simulink model "Sistema"  (R2023a)
settings: Solver=ode15s  StartTime=0.0  StopTime=10.0  MaxStep=1E-3  RelTol=1e-3
libraries: fl_lib x21, nesl_utility x9, slpidlib x2
settings Model: Creator=lunit  LastModifiedBy=Dino
settings DataIOCC: SaveFormat=Array  ReturnWorkspaceOutputs=off  TimeSaveName=t
settings DebuggingCC: AlgebraicLoopMsg=none  ArtificialAlgebraicLoopMsg=none  MaxConsecutiveZCsMsg=none  UnconnectedInputMsg=warning  UnconnectedOutputMsg=warning  UnconnectedLineMsg=warning  ModelReferenceExtraNoncontSigs=none  OperatingPointInterfaceChecksumMismatchMsg=none
settings ModelReferenceCC: EnableRefExpFcnMdlSchedulingChecks=on
settings RTWCC: DLArmComputeVersion=19.05

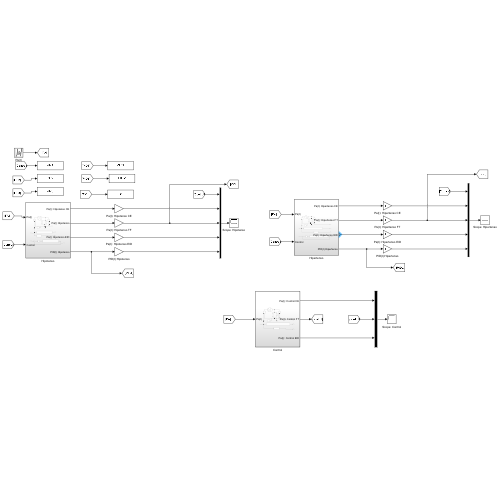
[thumbnail: Simulink's stored preview of the top-level diagram]
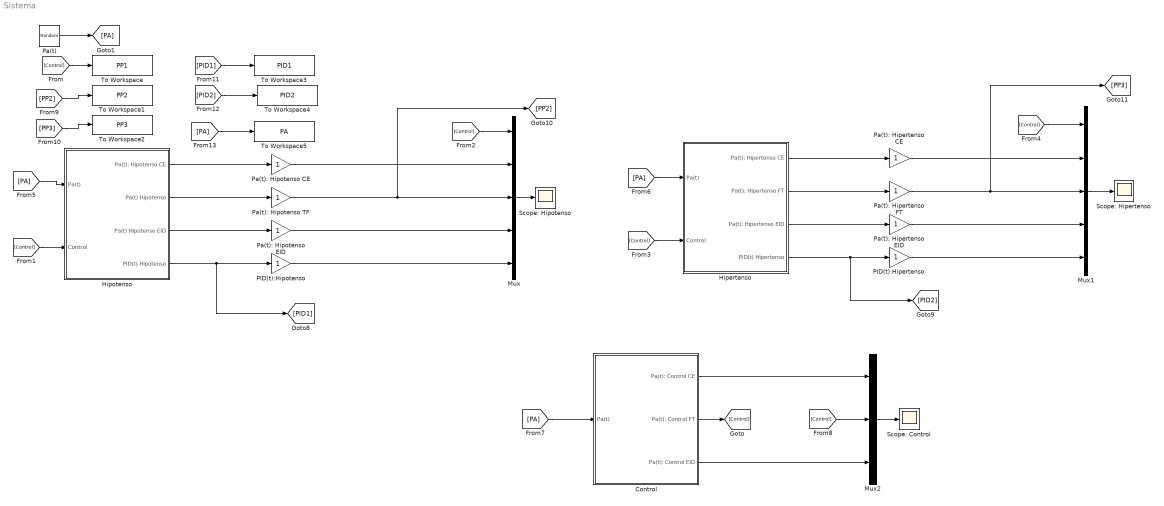
== system Sistema ==
  Control : Subsystem
  Hipertenso : Subsystem
  Hipotenso : Subsystem
  Mux : Mux  Inputs=5
  Mux1 : Mux  Inputs=5
  Mux2 : Mux  Inputs=3
  PID(t):Hipertenso : Gain
  PID(t):Hipotenso : Gain
  Pa(t) : UniformRandomNumber  Minimum=-0.2  Seed=106  SampleTime=0.5
  Pa(t): Hipertenso CE : Gain
  Pa(t): Hipertenso EID : Gain
  Pa(t): Hipertenso FT : Gain
  Pa(t): Hipotenso CE : Gain
  Pa(t): Hipotenso EID : Gain
  Pa(t): Hipotenso TF : Gain
  Scope: Control : Scope
  Scope: Hipertenso : Scope
  Scope: Hipotenso : Scope
  To Workspace : ToWorkspace  VariableName=PP1  SampleTime=-1
  To Workspace1 : ToWorkspace  VariableName=PP2  SampleTime=-1
  To Workspace2 : ToWorkspace  VariableName=PP3  SampleTime=-1
  To Workspace3 : ToWorkspace  VariableName=PID1  SampleTime=-1
  To Workspace4 : ToWorkspace  VariableName=PID2  SampleTime=-1
  To Workspace5 : ToWorkspace  VariableName=PA  SampleTime=-1
  wires:
  Mux/1 -> Scope: Hipotenso/1
  Hipotenso/1(Pa(t): Hipotenso CE) -> Pa(t): Hipotenso CE/1
  Hipotenso/2(Pa(t) Hipotenso) -> Pa(t): Hipotenso TF/1
  Hipotenso/3(Pa(t) Hipotenso EID) -> Pa(t): Hipotenso EID/1
  Hipotenso/4(PID(t) Hipotenso) -> [PID1], PID(t):Hipotenso/1
  [Control] -> Mux/1
  Pa(t): Hipotenso CE/1 -> Mux/2
  PID(t):Hipotenso/1 -> Mux/5
  Pa(t): Hipotenso EID/1 -> Mux/4
  Pa(t): Hipotenso TF/1 -> [PP2], Mux/3
  [Control] -> Hipotenso/2(Control)
  Pa(t): Hipertenso FT/1 -> [PP3], Mux1/3
  PID(t):Hipertenso/1 -> Mux1/5
  Mux1/1 -> Scope: Hipertenso/1
  Hipertenso/3(Pa(t): Hipertenso EID) -> Pa(t): Hipertenso EID/1
  Hipertenso/1(Pa(t): Hipertenso CE) -> Pa(t): Hipertenso CE/1
  Hipertenso/4(PID(t) Hipertenso) -> [PID2], PID(t):Hipertenso/1
  Pa(t): Hipertenso CE/1 -> Mux1/2
  Pa(t): Hipertenso EID/1 -> Mux1/4
  [Control] -> Mux1/1
  Hipertenso/2(Pa(t): Hipertenso FT) -> Pa(t): Hipertenso FT/1
  [Control] -> Hipertenso/2(Control)
  Pa(t)/1 -> [PA]
  [PA] -> Hipotenso/1(Pa(t))
  [PA] -> Hipertenso/1(Pa(t))
  Control/2(Pa(t): Control FT) -> [Control]
  [PA] -> Control/1(Pa(t))
  Mux2/1 -> Scope: Control/1
  Control/3(Pa(t): Control EID) -> Mux2/3
  Control/1(Pa(t): Control CE) -> Mux2/1
  [Control] -> Mux2/2
  [Control] -> To Workspace/1
  [PP2] -> To Workspace1/1
  [PP3] -> To Workspace2/1
  [PID1] -> To Workspace3/1
  [PID2] -> To Workspace4/1
  [PA] -> To Workspace5/1

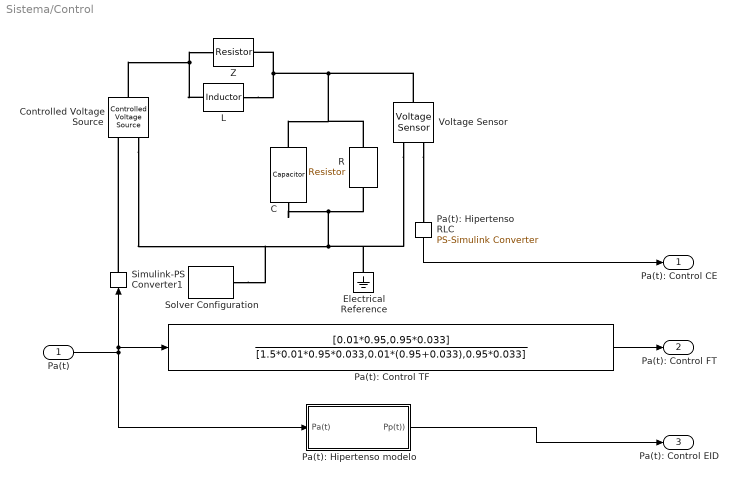
== system Sistema/Control ==
  Pa(t) : Inport
  C : fl_lib/Electrical/Electrical Elements/Capacitor  c=1.5 F  r=1e-6 Ohm  g=0 1/Ohm  i_specify=off  i_priority=None  i=0 A  i_nominal_specify=off  i_nominal_unit=A  i_nominal_value=1  v_specify=off  v_priority=None  v=0 V  v_nominal_specify=off  v_nominal_unit=V  v_nominal_value=1  vc_specify=off  vc_priority=High  vc=0 V  vc_nominal_specify=off  vc_nominal_unit=V  vc_nominal_value=1
  Controlled Voltage Source : fl_lib/Electrical/Electrical Sources/Controlled Voltage Source
  Electrical Reference : fl_lib/Electrical/Electrical Elements/Electrical Reference
  L : fl_lib/Electrical/Electrical Elements/Inductor  l=0.01 H  r=0 Ohm  g=1e-9 1/Ohm  i_specify=off  i_priority=None  i=0 A  i_nominal_specify=off  i_nominal_unit=A  i_nominal_value=1  v_specify=off  v_priority=None  v=0 V  v_nominal_specify=off  v_nominal_unit=V  v_nominal_value=1  i_L_specify=off  i_L_priority=High  i_L=0 A  i_L_nominal_specify=off  i_L_nominal_unit=A  i_L_nominal_value=1
  Pa(t): Control TF : TransferFcn  Numerator=[0.01*0.95,0.95*0.033]  Denominator=[1.5*0.01*0.95*0.033,0.01*(0.95+0.033),0.95*0.033]
  Pa(t): Hipertenso RLC : nesl_utility/PS-Simulink Converter  PhysicalDomain=network_engine_domain  SubClassName=ps_output  LeftPortType=input  RightPortType=output  PseudoPeriodic=off  Frequencies=[]  VectorFormat=1-D array  Unit=inherit  AffineConversion=off
  Pa(t): Hipertenso modelo : Subsystem
  R : fl_lib/Electrical/Electrical Elements/Resistor  R=0.95 Ohm  i_specify=off  i_priority=None  i=0 A  i_nominal_specify=off  i_nominal_unit=A  i_nominal_value=1  v_specify=off  v_priority=None  v=0 V  v_nominal_specify=off  v_nominal_unit=V  v_nominal_value=1
  Simulink-PS Converter1 : nesl_utility/Simulink-PS Converter  PhysicalDomain=network_engine_domain  SubClassName=ps_input  LeftPortType=input  RightPortType=output  PseudoPeriodic=off  Frequencies=[]  NoiseDistribution=none  NoiseParameters=[]  Unit=1  AffineConversion=off  FilteringAndDerivatives=provide  SimscapeFilterOrder=1  InputFilterTimeConstant=0.001  UdotUserProvided=0
  Solver Configuration : nesl_utility/Solver Configuration  PhysicalDomain=network_engine_domain  SubClassName=solver  LeftPortType=input  RightPortType=generic  Tones=[]  Harmonics=[]  SimulateNoise=off  Profile=off  UseLocalSampling=off  EnableSwitchedLinearOptims=on  FrequencyDomain=off  UseCCode=off  RelTol=0.001  AbsTol=1e-06  MinStep=1e-09  ToWorkspace=off  RevertToSquareIcSolve=off  NumHomotopyIterations=100  PhasorMode=off  PhasorModeNumHarmonics=1  ConsistencySolver=NEWTON_FTOL  IndexReductionMethod=DerivativeReplacement  DoDC=off  ResidualTolerance=1e-09  ConsistencyTolSource=GLOBAL  ConsistencyAbsTol=0.001  ConsistencyRelTol=0.001  ConsistencyTolFactor=0.001  UseLocalSolver=off  LocalSolverChoice=NE_BACKWARD_EULER_ADVANCER  ResolveIndetEquations=on  FunctionEvalNumThread=1  LocalSolverSampleTime=0.001  DoFixedCost=off  MaxNonlinIter=3  MaxModeIter=2  ComputeImpulses=off  ImpulseIterations=2  LinearAlgebra=auto  LinearAlgebraNumThread=0  EquationFormulation=NE_TIME_EF  DelaysMemoryBudget=1024  AutomaticFiltering=on  FilteringTimeConstant=0.001  PartitionStorageMethod=AS_NEEDED  PartitionMemoryBudget=1024  PartitionMethod=ROBUST
  Voltage Sensor : fl_lib/Electrical/Electrical Sensors/Voltage Sensor
  Z : fl_lib/Electrical/Electrical Elements/Resistor  R=0.033 Ohm  i_specify=off  i_priority=None  i=0 A  i_nominal_specify=off  i_nominal_unit=A  i_nominal_value=1  v_specify=off  v_priority=None  v=0 V  v_nominal_specify=off  v_nominal_unit=V  v_nominal_value=1
  Pa(t): Control CE : Outport
  Pa(t): Control FT : Outport  Port=2
  Pa(t): Control EID : Outport  Port=3
  wires:
  Pa(t)/1 -> Pa(t): Hipertenso modelo/1(Pa(t)), Pa(t): Control TF/1, Simulink-PS Converter1/1
  Pa(t): Hipertenso RLC/1 -> Pa(t): Control CE/1
  Pa(t): Hipertenso modelo/1(Pp(t))) -> Pa(t): Control EID/1
  Pa(t): Control TF/1 -> Pa(t): Control FT/1
  connections:
  Voltage Sensor/RConn1 -- Pa(t): Hipertenso RLC/LConn1
  Simulink-PS Converter1/RConn1 -- Controlled Voltage Source/RConn1
  Controlled Voltage Source/LConn1 -- L/LConn1 -- Z/LConn1
  L/RConn1 -- Z/RConn1 -- Voltage Sensor/LConn1 -- R/LConn1 -- C/LConn1
  C/RConn1 -- Electrical Reference/LConn1 -- Voltage Sensor/RConn2 -- Controlled Voltage Source/RConn2 -- Solver Configuration/RConn1 -- R/RConn1

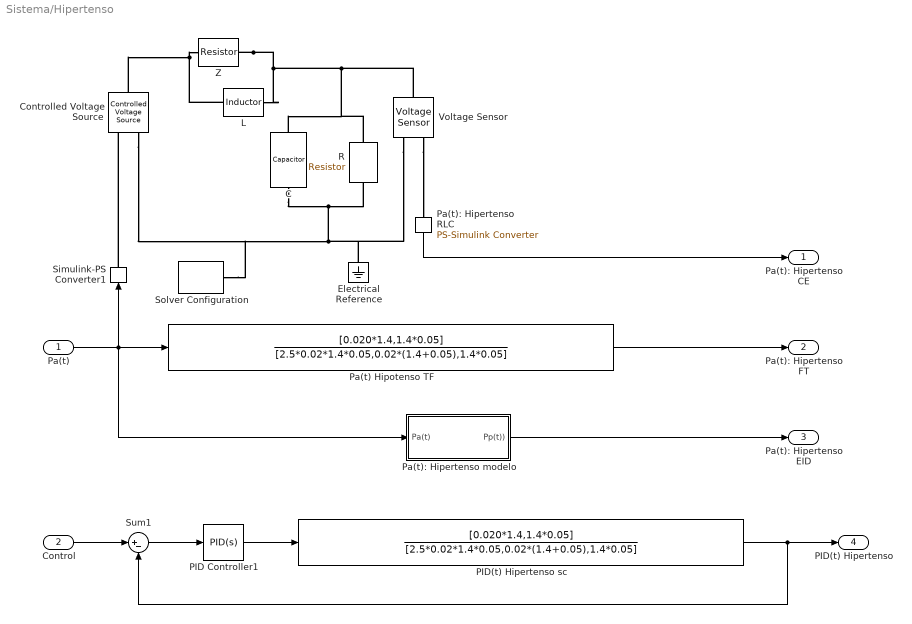
== system Sistema/Hipertenso ==
  Pa(t) : Inport
  Control : Inport  Port=2
  C : fl_lib/Electrical/Electrical Elements/Capacitor  c=2.5 F  r=1e-6 Ohm  g=0 1/Ohm  i_specify=off  i_priority=None  i=0 A  i_nominal_specify=off  i_nominal_unit=A  i_nominal_value=1  v_specify=off  v_priority=None  v=0 V  v_nominal_specify=off  v_nominal_unit=V  v_nominal_value=1  vc_specify=off  vc_priority=High  vc=0 V  vc_nominal_specify=off  vc_nominal_unit=V  vc_nominal_value=1
  Controlled Voltage Source : fl_lib/Electrical/Electrical Sources/Controlled Voltage Source
  Electrical Reference : fl_lib/Electrical/Electrical Elements/Electrical Reference
  L : fl_lib/Electrical/Electrical Elements/Inductor  l=0.02 H  r=0 Ohm  g=1e-9 1/Ohm  i_specify=off  i_priority=None  i=0 A  i_nominal_specify=off  i_nominal_unit=A  i_nominal_value=1  v_specify=off  v_priority=None  v=0 V  v_nominal_specify=off  v_nominal_unit=V  v_nominal_value=1  i_L_specify=off  i_L_priority=High  i_L=0 A  i_L_nominal_specify=off  i_L_nominal_unit=A  i_L_nominal_value=1
  PID Controller1 : slpidlib/PID Controller  Controller=PID  Form=Parallel  TimeDomain=Continuous-time  UseExternalTs=off  SampleTime=-1  IntegratorMethod=Forward Euler  FilterMethod=Forward Euler  ControllerParametersSource=internal  P=5.71697910151292  I=98.3466226969931  UseKiTs=off  D=0.0309945192714663  N=88.3932329939867  UseFilter=on  TunerSelectOption=Transfer Function Based (PID Tuner App)  InitialConditionSource=internal  InitialConditionForIntegrator=0  InitialConditionForFilter=0  DifferentiatorICPrevScaledInput=0  ExternalReset=none  TrackingMode=off  Kt=1  LimitOutput=off  SatLimitsSource=internal  UpperSaturationLimit=inf  LowerSaturationLimit=-inf  LinearizeAsGain=on  AntiWindupMode=none  Kb=1  LimitIntegrator=off  UpperIntegratorSaturationLimit=inf  LowerIntegratorSaturationLimit=-inf  POutMin=[]  POutMax=[]  IOutMin=[]  IOutMax=[]  DOutMin=[]  DOutMax=[]  NOutMin=[]  NOutMax=[]  SumOutMin=[]  SumOutMax=[]  SaturationOutMin=[]  SaturationOutMax=[]  PParamMin=[]  PParamMax=[]  IParamMin=[]  IParamMax=[]  DParamMin=[]  DParamMax=[]  NParamMin=[]  NParamMax=[]  KbParamMin=[]  KbParamMax=[]  KtParamMin=[]  KtParamMax=[]  KbOutMin=[]  KbOutMax=[]  KtOutMin=[]  KtOutMax=[]  IntegratorOutMin=[]  IntegratorOutMax=[]  FilterOutMin=[]  FilterOutMax=[]  SumI1OutMin=[]  SumI1OutMax=[]  SumI2OutMin=[]  SumI2OutMax=[]  SumI3OutMin=[]  SumI3OutMax=[]  SumI4OutMin=[]  SumI4OutMax=[]  SumDOutMin=[]  SumDOutMax=[]  DifferentiatorOutMin=[]  DifferentiatorOutMax=[]  FilterDiffOutCoefMin=[]  FilterDiffOutCoefMax=[]  ReciprocalOutMin=[]  ReciprocalOutMax=[]  SumDenOutMin=[]  SumDenOutMax=[]  SumNumOutMin=[]  SumNumOutMax=[]  DivideOutMin=[]  DivideOutMax=[]  UdiffTsProdOutMin=[]  UdiffTsProdOutMax=[]  NTsProdOutMin=[]  NTsProdOutMax=[]  UintegralTsProdOutMin=[]  UintegralTsProdOutMax=[]  UngainTsProdOutMin=[]  UngainTsProdOutMax=[]  ClampingZeroOutDataTypeStr=Inherit: Inherit via back propagation  ClampingZeroOutMin=[]  ClampingZeroOutMax=[]  FilterDenConstantOutDataTypeStr=Inherit: Inherit via back propagation  FilterDenConstantOutMin=[]  FilterDenConstantOutMax=[]  PCopyOutDataTypeStr=Inherit: Inherit via back propagation  PCopyOutMin=[]  PCopyOutMax=[]  NCopyOutDataTypeStr=Inherit: Inherit via back propagation  NCopyOutMin=[]  NCopyOutMax=[]  IntegratorContinuousStateAttributes=''  IntegratorStateMustResolveToSignalObject=off  IntegratorRTWStateStorageClass=Auto  FilterContinuousStateAttributes=''  FilterStateMustResolveToSignalObject=off  FilterRTWStateStorageClass=Auto  ParallelPVariant=InternalParameters  IdealPVariant=Disabled  IVariant=InternalParameters  DVariant=InternalParameters  IntegratorVariant=Continuous  SatVariant=Disabled  AWVariant=Passthrough  PCopyVariant=Disabled  TRVariant=Disabled  FdbkBlocksVariant=Forward  IdealPFdbkVariant=Disabled  SatFdbkVariant=Disabled  DerivativeFilterVariant=ContFilter  NVariant=InternalParameters  NCopyVariant=Disabled  FilterICVariant=InternalICsFilter  IntegratorICVariant=InternalICs  ExternalResetVariant=Disabled  TRSumVariant=Passthrough  SumFdbkVariant=Disabled  SumVariant=Sum_PID  TsampFilterVariant=InternalTs  TsampNgainVariant=Passthrough  TsampIntegralVariant=Disabled_SignalSpec  ExternalSaturationOutDataTypeStr=Inherit: Same as second input
  PID(t) Hipertenso sc : TransferFcn  Numerator=[0.020*1.4,1.4*0.05]  Denominator=[2.5*0.02*1.4*0.05,0.02*(1.4+0.05),1.4*0.05]
  Pa(t) Hipotenso TF : TransferFcn  Numerator=[0.020*1.4,1.4*0.05]  Denominator=[2.5*0.02*1.4*0.05,0.02*(1.4+0.05),1.4*0.05]
  Pa(t): Hipertenso RLC : nesl_utility/PS-Simulink Converter  PhysicalDomain=network_engine_domain  SubClassName=ps_output  LeftPortType=input  RightPortType=output  PseudoPeriodic=off  Frequencies=[]  VectorFormat=1-D array  Unit=inherit  AffineConversion=off
  Pa(t): Hipertenso modelo : Subsystem
  R : fl_lib/Electrical/Electrical Elements/Resistor  R=1.4 Ohm  i_specify=off  i_priority=None  i=0 A  i_nominal_specify=off  i_nominal_unit=A  i_nominal_value=1  v_specify=off  v_priority=None  v=0 V  v_nominal_specify=off  v_nominal_unit=V  v_nominal_value=1
  Simulink-PS Converter1 : nesl_utility/Simulink-PS Converter  PhysicalDomain=network_engine_domain  SubClassName=ps_input  LeftPortType=input  RightPortType=output  PseudoPeriodic=off  Frequencies=[]  NoiseDistribution=none  NoiseParameters=[]  Unit=1  AffineConversion=off  FilteringAndDerivatives=provide  SimscapeFilterOrder=1  InputFilterTimeConstant=0.001  UdotUserProvided=0
  Solver Configuration : nesl_utility/Solver Configuration  PhysicalDomain=network_engine_domain  SubClassName=solver  LeftPortType=input  RightPortType=generic  Tones=[]  Harmonics=[]  SimulateNoise=off  Profile=off  UseLocalSampling=off  EnableSwitchedLinearOptims=on  FrequencyDomain=off  UseCCode=off  RelTol=0.001  AbsTol=1e-06  MinStep=1e-09  ToWorkspace=off  RevertToSquareIcSolve=off  NumHomotopyIterations=100  PhasorMode=off  PhasorModeNumHarmonics=1  ConsistencySolver=NEWTON_FTOL  IndexReductionMethod=DerivativeReplacement  DoDC=off  ResidualTolerance=1e-09  ConsistencyTolSource=GLOBAL  ConsistencyAbsTol=0.001  ConsistencyRelTol=0.001  ConsistencyTolFactor=0.001  UseLocalSolver=off  LocalSolverChoice=NE_BACKWARD_EULER_ADVANCER  ResolveIndetEquations=on  FunctionEvalNumThread=1  LocalSolverSampleTime=0.001  DoFixedCost=off  MaxNonlinIter=3  MaxModeIter=2  ComputeImpulses=off  ImpulseIterations=2  LinearAlgebra=auto  LinearAlgebraNumThread=0  EquationFormulation=NE_TIME_EF  DelaysMemoryBudget=1024  AutomaticFiltering=on  FilteringTimeConstant=0.001  PartitionStorageMethod=AS_NEEDED  PartitionMemoryBudget=1024  PartitionMethod=ROBUST
  Sum1 : Sum  Inputs=|+-
  Voltage Sensor : fl_lib/Electrical/Electrical Sensors/Voltage Sensor
  Z : fl_lib/Electrical/Electrical Elements/Resistor  R=0.05 Ohm  i_specify=off  i_priority=None  i=0 A  i_nominal_specify=off  i_nominal_unit=A  i_nominal_value=1  v_specify=off  v_priority=None  v=0 V  v_nominal_specify=off  v_nominal_unit=V  v_nominal_value=1
  Pa(t): Hipertenso CE : Outport
  Pa(t): Hipertenso FT : Outport  Port=2
  Pa(t): Hipertenso EID : Outport  Port=3
  PID(t) Hipertenso : Outport  Port=4
  wires:
  PID Controller1/1 -> PID(t) Hipertenso sc/1
  Sum1/1 -> PID Controller1/1
  PID(t) Hipertenso sc/1 -> Sum1/2, PID(t) Hipertenso/1
  Pa(t)/1 -> Pa(t) Hipotenso TF/1, Pa(t): Hipertenso modelo/1(Pa(t)), Simulink-PS Converter1/1
  Pa(t) Hipotenso TF/1 -> Pa(t): Hipertenso FT/1
  Pa(t): Hipertenso RLC/1 -> Pa(t): Hipertenso CE/1
  Control/1 -> Sum1/1
  Pa(t): Hipertenso modelo/1(Pp(t))) -> Pa(t): Hipertenso EID/1
  connections:
  Voltage Sensor/RConn1 -- Pa(t): Hipertenso RLC/LConn1
  Simulink-PS Converter1/RConn1 -- Controlled Voltage Source/RConn1
  Controlled Voltage Source/LConn1 -- L/LConn1 -- Z/LConn1
  Z/RConn1 -- L/RConn1 -- Voltage Sensor/LConn1 -- C/LConn1 -- R/LConn1
  C/RConn1 -- Electrical Reference/LConn1 -- Voltage Sensor/RConn2 -- Controlled Voltage Source/RConn2 -- Solver Configuration/RConn1 -- R/RConn1

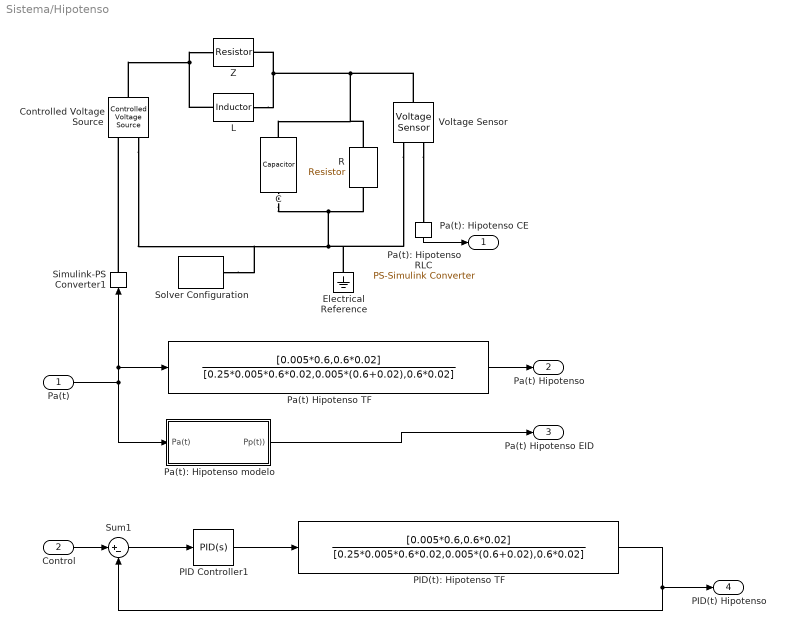
== system Sistema/Hipotenso ==
  Pa(t) : Inport
  Control : Inport  Port=2
  C : fl_lib/Electrical/Electrical Elements/Capacitor  c=0.25 F  r=1e-6 Ohm  g=0 1/Ohm  i_specify=off  i_priority=None  i=0 A  i_nominal_specify=off  i_nominal_unit=A  i_nominal_value=1  v_specify=off  v_priority=None  v=0 V  v_nominal_specify=off  v_nominal_unit=V  v_nominal_value=1  vc_specify=off  vc_priority=High  vc=0 V  vc_nominal_specify=off  vc_nominal_unit=V  vc_nominal_value=1
  Controlled Voltage Source : fl_lib/Electrical/Electrical Sources/Controlled Voltage Source
  Electrical Reference : fl_lib/Electrical/Electrical Elements/Electrical Reference
  L : fl_lib/Electrical/Electrical Elements/Inductor  l=0.005 H  r=0 Ohm  g=1e-9 1/Ohm  i_specify=off  i_priority=None  i=0 A  i_nominal_specify=off  i_nominal_unit=A  i_nominal_value=1  v_specify=off  v_priority=None  v=0 V  v_nominal_specify=off  v_nominal_unit=V  v_nominal_value=1  i_L_specify=off  i_L_priority=High  i_L=0 A  i_L_nominal_specify=off  i_L_nominal_unit=A  i_L_nominal_value=1
  PID Controller1 : slpidlib/PID Controller  Controller=PID  Form=Parallel  TimeDomain=Continuous-time  UseExternalTs=off  SampleTime=-1  IntegratorMethod=Forward Euler  FilterMethod=Forward Euler  ControllerParametersSource=internal  P=1.31715584559549  I=295.122019144814  UseKiTs=off  D=0.000356490864198976  N=467.636469275933  UseFilter=on  TunerSelectOption=Transfer Function Based (PID Tuner App)  InitialConditionSource=internal  InitialConditionForIntegrator=0  InitialConditionForFilter=0  DifferentiatorICPrevScaledInput=0  ExternalReset=none  TrackingMode=off  Kt=1  LimitOutput=off  SatLimitsSource=internal  UpperSaturationLimit=inf  LowerSaturationLimit=-inf  LinearizeAsGain=on  AntiWindupMode=none  Kb=1  LimitIntegrator=off  UpperIntegratorSaturationLimit=inf  LowerIntegratorSaturationLimit=-inf  POutMin=[]  POutMax=[]  IOutMin=[]  IOutMax=[]  DOutMin=[]  DOutMax=[]  NOutMin=[]  NOutMax=[]  SumOutMin=[]  SumOutMax=[]  SaturationOutMin=[]  SaturationOutMax=[]  PParamMin=[]  PParamMax=[]  IParamMin=[]  IParamMax=[]  DParamMin=[]  DParamMax=[]  NParamMin=[]  NParamMax=[]  KbParamMin=[]  KbParamMax=[]  KtParamMin=[]  KtParamMax=[]  KbOutMin=[]  KbOutMax=[]  KtOutMin=[]  KtOutMax=[]  IntegratorOutMin=[]  IntegratorOutMax=[]  FilterOutMin=[]  FilterOutMax=[]  SumI1OutMin=[]  SumI1OutMax=[]  SumI2OutMin=[]  SumI2OutMax=[]  SumI3OutMin=[]  SumI3OutMax=[]  SumI4OutMin=[]  SumI4OutMax=[]  SumDOutMin=[]  SumDOutMax=[]  DifferentiatorOutMin=[]  DifferentiatorOutMax=[]  FilterDiffOutCoefMin=[]  FilterDiffOutCoefMax=[]  ReciprocalOutMin=[]  ReciprocalOutMax=[]  SumDenOutMin=[]  SumDenOutMax=[]  SumNumOutMin=[]  SumNumOutMax=[]  DivideOutMin=[]  DivideOutMax=[]  UdiffTsProdOutMin=[]  UdiffTsProdOutMax=[]  NTsProdOutMin=[]  NTsProdOutMax=[]  UintegralTsProdOutMin=[]  UintegralTsProdOutMax=[]  UngainTsProdOutMin=[]  UngainTsProdOutMax=[]  ClampingZeroOutDataTypeStr=Inherit: Inherit via back propagation  ClampingZeroOutMin=[]  ClampingZeroOutMax=[]  FilterDenConstantOutDataTypeStr=Inherit: Inherit via back propagation  FilterDenConstantOutMin=[]  FilterDenConstantOutMax=[]  PCopyOutDataTypeStr=Inherit: Inherit via back propagation  PCopyOutMin=[]  PCopyOutMax=[]  NCopyOutDataTypeStr=Inherit: Inherit via back propagation  NCopyOutMin=[]  NCopyOutMax=[]  IntegratorContinuousStateAttributes=''  IntegratorStateMustResolveToSignalObject=off  IntegratorRTWStateStorageClass=Auto  FilterContinuousStateAttributes=''  FilterStateMustResolveToSignalObject=off  FilterRTWStateStorageClass=Auto  ParallelPVariant=InternalParameters  IdealPVariant=Disabled  IVariant=InternalParameters  DVariant=InternalParameters  IntegratorVariant=Continuous  SatVariant=Disabled  AWVariant=Passthrough  PCopyVariant=Disabled  TRVariant=Disabled  FdbkBlocksVariant=Forward  IdealPFdbkVariant=Disabled  SatFdbkVariant=Disabled  DerivativeFilterVariant=ContFilter  NVariant=InternalParameters  NCopyVariant=Disabled  FilterICVariant=InternalICsFilter  IntegratorICVariant=InternalICs  ExternalResetVariant=Disabled  TRSumVariant=Passthrough  SumFdbkVariant=Disabled  SumVariant=Sum_PID  TsampFilterVariant=InternalTs  TsampNgainVariant=Passthrough  TsampIntegralVariant=Disabled_SignalSpec  ExternalSaturationOutDataTypeStr=Inherit: Same as second input
  PID(t): Hipotenso TF : TransferFcn  Numerator=[0.005*0.6,0.6*0.02]  Denominator=[0.25*0.005*0.6*0.02,0.005*(0.6+0.02),0.6*0.02]
  Pa(t) Hipotenso TF : TransferFcn  Numerator=[0.005*0.6,0.6*0.02]  Denominator=[0.25*0.005*0.6*0.02,0.005*(0.6+0.02),0.6*0.02]
  Pa(t): Hipotenso RLC : nesl_utility/PS-Simulink Converter  PhysicalDomain=network_engine_domain  SubClassName=ps_output  LeftPortType=input  RightPortType=output  PseudoPeriodic=off  Frequencies=[]  VectorFormat=1-D array  Unit=inherit  AffineConversion=off
  Pa(t): Hipotenso modelo : Subsystem
  R : fl_lib/Electrical/Electrical Elements/Resistor  R=0.6 Ohm  i_specify=off  i_priority=None  i=0 A  i_nominal_specify=off  i_nominal_unit=A  i_nominal_value=1  v_specify=off  v_priority=None  v=0 V  v_nominal_specify=off  v_nominal_unit=V  v_nominal_value=1
  Simulink-PS Converter1 : nesl_utility/Simulink-PS Converter  PhysicalDomain=network_engine_domain  SubClassName=ps_input  LeftPortType=input  RightPortType=output  PseudoPeriodic=off  Frequencies=[]  NoiseDistribution=none  NoiseParameters=[]  Unit=1  AffineConversion=off  FilteringAndDerivatives=provide  SimscapeFilterOrder=1  InputFilterTimeConstant=0.001  UdotUserProvided=0
  Solver Configuration : nesl_utility/Solver Configuration  PhysicalDomain=network_engine_domain  SubClassName=solver  LeftPortType=input  RightPortType=generic  Tones=[]  Harmonics=[]  SimulateNoise=off  Profile=off  UseLocalSampling=off  EnableSwitchedLinearOptims=on  FrequencyDomain=off  UseCCode=off  RelTol=0.001  AbsTol=1e-06  MinStep=1e-09  ToWorkspace=off  RevertToSquareIcSolve=off  NumHomotopyIterations=100  PhasorMode=off  PhasorModeNumHarmonics=1  ConsistencySolver=NEWTON_FTOL  IndexReductionMethod=DerivativeReplacement  DoDC=off  ResidualTolerance=1e-09  ConsistencyTolSource=GLOBAL  ConsistencyAbsTol=0.001  ConsistencyRelTol=0.001  ConsistencyTolFactor=0.001  UseLocalSolver=off  LocalSolverChoice=NE_BACKWARD_EULER_ADVANCER  ResolveIndetEquations=on  FunctionEvalNumThread=1  LocalSolverSampleTime=0.001  DoFixedCost=off  MaxNonlinIter=3  MaxModeIter=2  ComputeImpulses=off  ImpulseIterations=2  LinearAlgebra=auto  LinearAlgebraNumThread=0  EquationFormulation=NE_TIME_EF  DelaysMemoryBudget=1024  AutomaticFiltering=on  FilteringTimeConstant=0.001  PartitionStorageMethod=AS_NEEDED  PartitionMemoryBudget=1024  PartitionMethod=ROBUST
  Sum1 : Sum  Inputs=|+-
  Voltage Sensor : fl_lib/Electrical/Electrical Sensors/Voltage Sensor
  Z : fl_lib/Electrical/Electrical Elements/Resistor  R=0.02 Ohm  i_specify=off  i_priority=None  i=0 A  i_nominal_specify=off  i_nominal_unit=A  i_nominal_value=1  v_specify=off  v_priority=None  v=0 V  v_nominal_specify=off  v_nominal_unit=V  v_nominal_value=1
  Pa(t): Hipotenso CE : Outport
  Pa(t) Hipotenso : Outport  Port=2
  Pa(t) Hipotenso EID : Outport  Port=3
  PID(t) Hipotenso : Outport  Port=4
  wires:
  PID Controller1/1 -> PID(t): Hipotenso TF/1
  Sum1/1 -> PID Controller1/1
  PID(t): Hipotenso TF/1 -> PID(t) Hipotenso/1, Sum1/2
  Pa(t)/1 -> Simulink-PS Converter1/1, Pa(t) Hipotenso TF/1, Pa(t): Hipotenso modelo/1(Pa(t))
  Pa(t) Hipotenso TF/1 -> Pa(t) Hipotenso/1
  Pa(t): Hipotenso RLC/1 -> Pa(t): Hipotenso CE/1
  Control/1 -> Sum1/1
  Pa(t): Hipotenso modelo/1(Pp(t))) -> Pa(t) Hipotenso EID/1
  connections:
  Voltage Sensor/RConn1 -- Pa(t): Hipotenso RLC/LConn1
  Simulink-PS Converter1/RConn1 -- Controlled Voltage Source/RConn1
  Controlled Voltage Source/LConn1 -- L/LConn1 -- Z/LConn1
  L/RConn1 -- Z/RConn1 -- Voltage Sensor/LConn1 -- C/LConn1 -- R/LConn1
  C/RConn1 -- Controlled Voltage Source/RConn2 -- Solver Configuration/RConn1 -- Electrical Reference/LConn1 -- Voltage Sensor/RConn2 -- R/RConn1

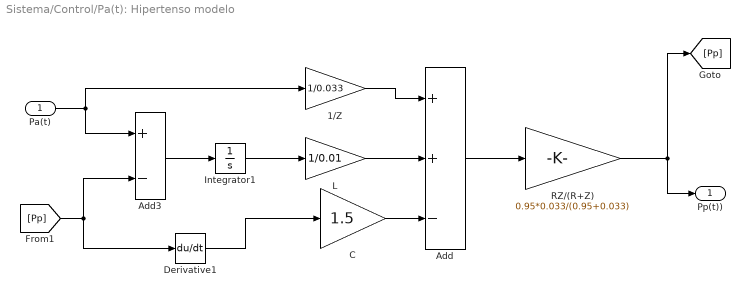
== system Sistema/Control/Pa(t): Hipertenso modelo ==
  Pa(t) : Inport
  1/Z : Gain  Gain=1/0.033
  Add : Sum  Inputs=++-
  Add3 : Sum  Inputs=+-
  C : Gain  Gain=1.5
  Derivative1 : Derivative
  Integrator1 : Integrator
  L : Gain  Gain=1/0.01
  RZ/(R+Z) : Gain  Gain=0.95*0.033/(0.95+0.033)
  Pp(t)) : Outport
  wires:
  Add/1 -> RZ/(R+Z)/1
  L/1 -> Add/2
  Pa(t)/1 -> 1/Z/1, Add3/1
  1/Z/1 -> Add/1
  Integrator1/1 -> L/1
  Add3/1 -> Integrator1/1
  C/1 -> Add/3
  Derivative1/1 -> C/1
  RZ/(R+Z)/1 -> [Pp], Pp(t))/1
  [Pp] -> Add3/2, Derivative1/1

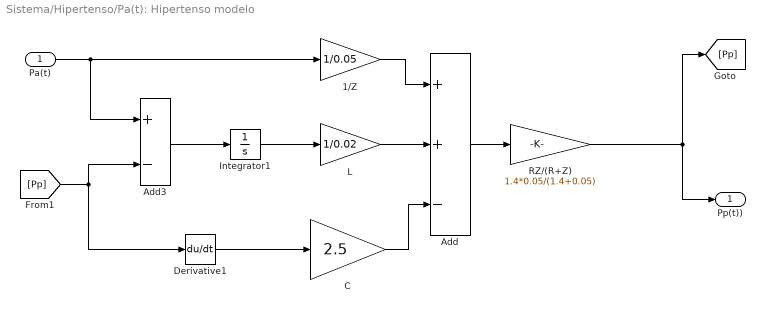
== system Sistema/Hipertenso/Pa(t): Hipertenso modelo ==
  Pa(t) : Inport
  1/Z : Gain  Gain=1/0.05
  Add : Sum  Inputs=++-
  Add3 : Sum  Inputs=+-
  C : Gain  Gain=2.5
  Derivative1 : Derivative
  Integrator1 : Integrator
  L : Gain  Gain=1/0.02
  RZ/(R+Z) : Gain  Gain=1.4*0.05/(1.4+0.05)
  Pp(t)) : Outport
  wires:
  Add/1 -> RZ/(R+Z)/1
  L/1 -> Add/2
  Pa(t)/1 -> Add3/1, 1/Z/1
  1/Z/1 -> Add/1
  Integrator1/1 -> L/1
  Add3/1 -> Integrator1/1
  C/1 -> Add/3
  Derivative1/1 -> C/1
  RZ/(R+Z)/1 -> [Pp], Pp(t))/1
  [Pp] -> Derivative1/1, Add3/2

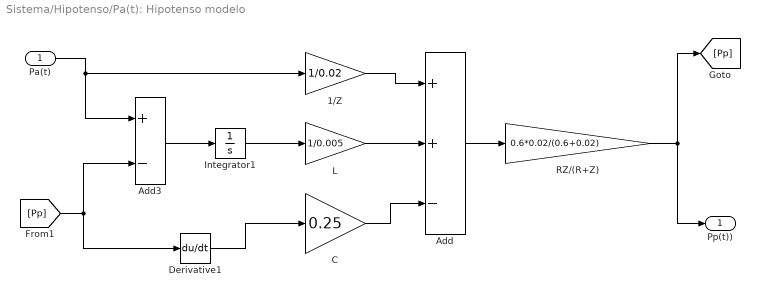
== system Sistema/Hipotenso/Pa(t): Hipotenso modelo ==
  Pa(t) : Inport
  1/Z : Gain  Gain=1/0.02
  Add : Sum  Inputs=++-
  Add3 : Sum  Inputs=+-
  C : Gain  Gain=0.25
  Derivative1 : Derivative
  Integrator1 : Integrator
  L : Gain  Gain=1/0.005
  RZ/(R+Z) : Gain  Gain=0.6*0.02/(0.6+0.02)
  Pp(t)) : Outport
  wires:
  Add/1 -> RZ/(R+Z)/1
  L/1 -> Add/2
  Pa(t)/1 -> Add3/1, 1/Z/1
  1/Z/1 -> Add/1
  Integrator1/1 -> L/1
  Add3/1 -> Integrator1/1
  C/1 -> Add/3
  Derivative1/1 -> C/1
  RZ/(R+Z)/1 -> [Pp], Pp(t))/1
  [Pp] -> Add3/2, Derivative1/1
